simulink model "mechanical_model"  (R2024b)
settings: Solver=VariableStepAuto  StartTime=0.0  StopTime=10.0  RelTol=1e-3
settings Model: Creator=rocke  LastModifiedBy=rocke

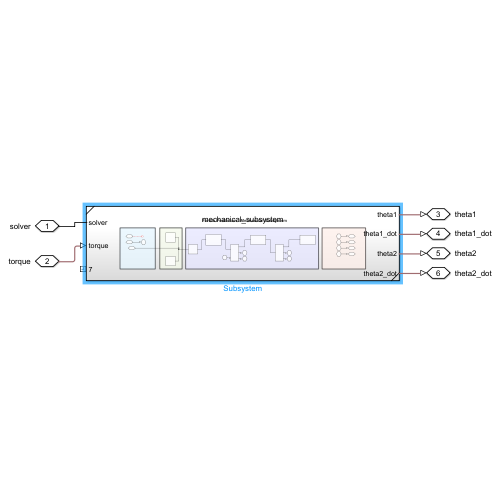
[thumbnail: Simulink's stored preview of the top-level diagram]
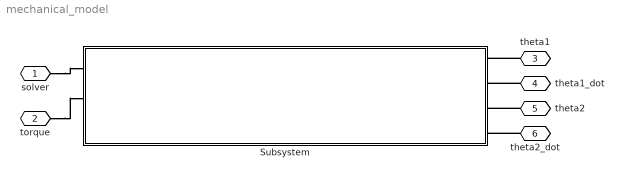
== system mechanical_model ==
  Subsystem : Subsystem  ReferencedSubsystem=mechanical_subsystem
  solver : PMIOPort  Side=Left
  torque : PMIOPort  Port=2  Side=Left
  theta1 : PMIOPort  Port=3  Side=Right
  theta1_dot : PMIOPort  Port=4  Side=Right
  theta2 : PMIOPort  Port=5  Side=Right
  theta2_dot : PMIOPort  Port=6  Side=Right
  connections:
  solver/RConn1 -- Subsystem/LConn1
  torque/RConn1 -- Subsystem/LConn2
  theta1/RConn1 -- Subsystem/RConn1
  theta1_dot/RConn1 -- Subsystem/RConn2
  theta2/RConn1 -- Subsystem/RConn3
  theta2_dot/RConn1 -- Subsystem/RConn4
